simulink model "voice_control_model2"  (R2021a)
settings: Solver=VariableStepAuto  StartTime=0.0  StopTime=30  RelTol=1e-3
settings Model: Creator=egwuo  LastModifiedBy=egwuo

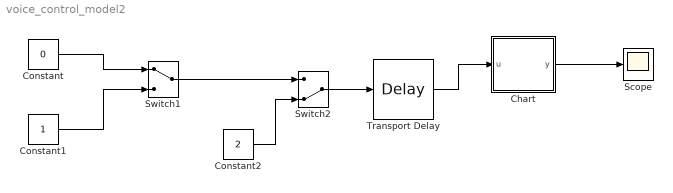
== system voice_control_model2 ==
  " Switch1" : ManualSwitch
  " Switch2" : ManualSwitch  CurrentSetting=0
  Chart : Stateflow chart  TreatAsAtomicUnit=on
  Constant : Constant  Value=0
  Constant1 : Constant
  Constant2 : Constant  Value=2
  Scope : Scope
  Transport Delay : TransportDelay  DelayTime=2
  wires:
  Chart/1(y) -> Scope/1
  Transport Delay/1 -> Chart/1(u)
  " Switch2"/1 -> Transport Delay/1
  Constant2/1 -> " Switch2"/2
  " Switch1"/1 -> " Switch2"/1
  Constant/1 -> " Switch1"/1
  Constant1/1 -> " Switch1"/2

== stateflow chart voice_control_model2/Chart ==
  state Idle
    y=0
  state FanOn
    y=1
  state LightOn
    y=2
  (default) -> Idle
  Idle -> LightOn [order 2] : [u == 2]
  Idle -> FanOn [order 1] : [u == 1]
  FanOn -> Idle : [u == 0]
  LightOn -> Idle : [u == 0]
  data: u input; y output
